simulink model "heli_q8"  (R2015b)
settings: Solver=ode1  StartTime=0.0  StopTime=inf  FixedStep=0.002  RelTol=1e-3
PostLoadFcn:
  | qc_set_target_type(getConfigSet(bdroot, 'QUARC Default Target Configuration'));
values from neighbouring files (symbols this model uses):
  F_aug = inv(C*inv(B*K_aug_K1-A)*B)    [init_heli.m]
  Joystick_gain_x = 1    [init_heli.m]
  Joystick_gain_y = 1    [init_heli.m]
  k_1 = k_f/(2*m_p*l_p)    (= 0.514757969303)    [init_heli.m]
  k_2 = (l_h*k_f)/(m_c*l_c^2+2*m_p*l_h^2)    (= 0.0828365392735)    [init_heli.m]
  k_3 = (v_s0*l_h*k_f)/(m_c*l_c^2+2*m_p*(l_h^2+l_p^2))    (= 0.611739028763)    [init_heli.m]
  K_aug = lqr(A_aug,B_aug,Q_aug,R_aug)    [init_heli.m]
  k_pd = (2*zeta*omega_0)/k_1    (= 7.77064220183)    [init_heli.m]
  k_pp = omega_0^2/k_1    (= 7.77064220183)    [init_heli.m]
  v_s0 = 7.7    [init_heli.m]
undefined symbols (not defined in the file or in its folder): HIL, qc_get_step_size
libraries: quarc_library x4, simulink x1
settings Model: SimulationMode=external  ExtModeTrigDuration=5000  Creator=Rchan  LastModifiedBy=torsteoe
settings SolverCC: PositivePriorityOrder=on
settings DataIOCC: SaveFormat=Array  SignalLoggingSaveFormat=ModelDataLogs
settings OptimizationCC: ExpressionDepthLimit=2147483647  InitFltsAndDblsToZero=on
settings DebuggingCC: SaveWithParameterizedLinksMsg=none  UnderspecifiedInitializationDetection=Classic  MergeDetectMultiDrivingBlocksExec=none  SolverPrmCheckMsg=warning  MultiTaskDSMMsg=warning  MultiTaskCondExecSysMsg=none  FcnCallInpInsideContextMsg=UseLocalSettings  StateNameClashWarn=warning
settings HardwareCC: ProdBitPerPointer=32  ProdLargestAtomicFloat=None  ProdIntDivRoundTo=Undefined  ProdEndianess=Unspecified  ProdWordSize=32  ProdHWDeviceType=32-bit Generic
settings RTWCC: SystemTargetFile=quarc_win64.tlc  TemplateMakefile=quarc_default_tmf  Description=QUARC Win64 Target
settings GRTTargetCC: ParMdlRefBuildCompliant=off  CompOptLevelCompliant=off  GeneratePreprocessorConditionals=Disable all  CombineOutputUpdateFcns=off  MatFileLogging=off  GRTInterface=on  UseToolchainInfoCompliant=off  ExtMode=on  ExtModeMexFile=quarc_comm
settings ConfigComp: CovModelRefEnable=Off  CovSFcnEnable=off

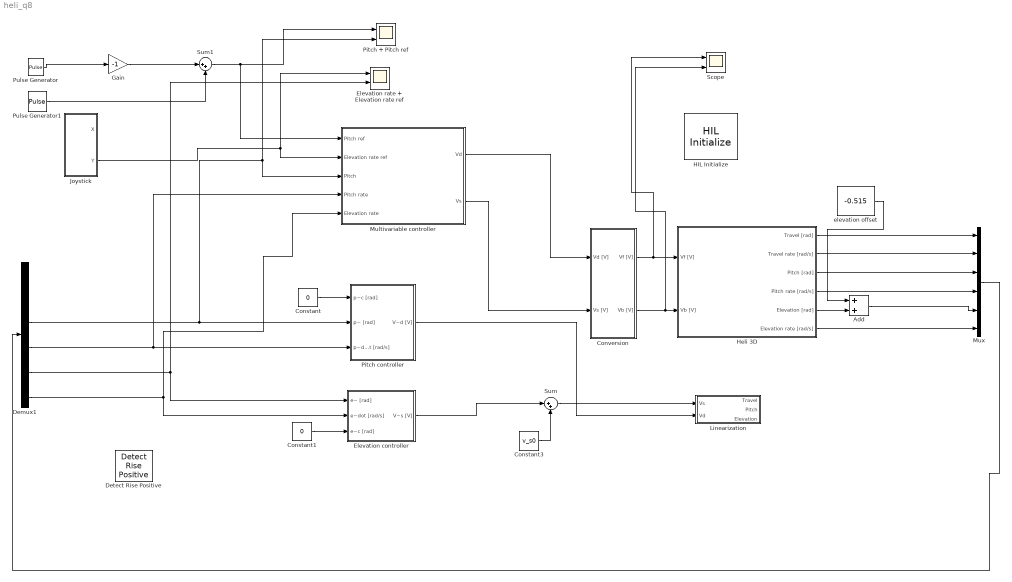
== system heli_q8 ==
  Add : Sum
  Constant : Constant  Value=0
  Constant1 : Constant  Value=0
  Constant3 : Constant  Value=v_s0
  Conversion : Subsystem
  Demux1 : Demux  Outputs=6
  Detect Rise Positive : simulink/Logic and Bit Operations/Detect Rise Positive  vinit=0  InputProcessing=Inherited  OutDataTypeStr=boolean
  Elevation controller : Subsystem
  Elevation rate + Elevation rate ref : Scope  NumInputPorts=2
  Gain : Gain  Gain=-1
  HIL Initialize : quarc_library/Data Acquisition/Generic/Configuration/HIL Initialize  Priority=-99  object_name=HIL-1  board_type=q8_usb  board_number=0  board_options=update_rate=normal;decimation=1  exclusive=off  active=off  hardware_clocks=[0:2]  clock_modes=[]  initial_clock_frequencies=[]  set_clock_params_at_start=off  set_clock_params_at_switch_in=off  set_clock_frequencies_at_start=off  set_clock_frequencies_at_switch_in=off  analog_input_channels=[0:7]  analog_input_maximums=10  analog_input_minimums=-10  set_analog_input_params_at_start=on  set_analog_input_params_at_switch_in=off  analog_output_channels=[0:7]  analog_output_maximums=10  analog_output_minimums=-10  initial_analog_outputs=[0]  final_analog_outputs=[0]  watchdog_analog_outputs=0  set_analog_output_params_at_start=on  set_analog_output_params_at_switch_in=off  set_analog_outputs_at_start=on  set_analog_outputs_at_switch_in=off  set_analog_outputs_at_terminate=on  set_analog_outputs_at_switch_out=off  set_analog_outputs_on_watchdog=off  digital_input_channels=[]  digital_output_channels=[]  digital_output_configuration=[]  initial_digital_outputs=[1]  final_digital_outputs=[1]  watchdog_digital_outputs=[1]  set_digital_output_params_at_start=off  set_digital_output_params_at_switch_in=off  set_digital_outputs_at_start=on  set_digital_outputs_at_switch_in=off  set_digital_outputs_at_terminate=on  set_digital_outputs_at_switch_out=off  set_digital_outputs_on_watchdog=off  encoder_channels=[0:7]  quadrature=[4]  encoder_filter_frequency=[]  initial_encoder_counts=[0]  set_encoder_params_at_start=on  set_encoder_params_at_switch_in=off  set_encoder_counts_at_start=on  set_encoder_counts_at_switch_in=off  pwm_channels=[0:7]  pwm_modes=0  pwm_frequency=99.532799999999995e6/4095  pwm_configuration=[0]  pwm_alignment=[0]  pwm_polarity=[1]  pwm_leading_deadband=[0]  pwm_trailing_deadband=[0]  initial_pwm_outputs=[0]  final_pwm_outputs=[0]  watchdog_pwm_outputs=[0]  set_pwm_params_at_start=on  set_pwm_params_at_switch_in=off  set_pwm_outputs_at_start=on  set_pwm_outputs_at_switch_in=off  set_pwm_outputs_at_terminate=on  set_pwm_outputs_at_switch_out=off  set_pwm_outputs_on_watchdog=off  other_output_channels=[]  initial_other_outputs=[]  final_other_outputs=[]  watchdog_other_outputs=[]  set_other_outputs_at_start=off  set_other_outputs_at_switch_in=off  set_other_outputs_at_terminate=off  set_other_outputs_at_switch_out=off  set_other_outputs_on_watchdog=off
  Heli 3D : Subsystem
  Joystick : Subsystem
  Linearization : Subsystem
  Multivariable controller : Subsystem
  Mux : Mux  Inputs=6
  Pitch + Pitch ref : Scope  NumInputPorts=2
  Pitch controller : Subsystem
  Pulse Generator : DiscretePulseGenerator  PulseType=Time based  Amplitude=0.5  Period=40  PulseWidth=50  PhaseDelay=10
  Pulse Generator1 : DiscretePulseGenerator  PulseType=Time based  Amplitude=0.5  Period=40  PulseWidth=50  PhaseDelay=30
  Scope : Scope  NumInputPorts=2
  Sum : Sum  Inputs=|++
  Sum1 : Sum  Inputs=|++
  elevation offset : Constant  Value=-0.515
  wires:
  Conversion/1(Vf [V]) -> Scope/1, Heli 3D/1(Vf [V])
  Heli 3D/1(Travel [rad]) -> Mux/1
  Heli 3D/2(Travel rate [rad/s]) -> Mux/2
  Heli 3D/3(Pitch [rad]) -> Mux/3
  Heli 3D/4(Pitch rate [rad/s]) -> Mux/4
  Heli 3D/5(Elevation [rad]) -> Add/2
  Heli 3D/6(Elevation rate [rad/s]) -> Mux/6
  Add/1 -> Mux/5
  elevation offset/1 -> Add/1
  Conversion/2(Vb [V]) -> Scope/2, Heli 3D/2(Vb [V])
  Constant/1 -> Pitch controller/1(p~c [rad])
  Constant1/1 -> Elevation controller/3(e~c [rad])
  Elevation controller/1(V~s [V]) -> Sum/1
  Sum/1 -> Linearization/1("Vs ")
  Pitch controller/1(V~d [V]) -> Linearization/2("Vd ")
  Joystick/2(Y) -> Elevation rate + Elevation rate ref/1, Multivariable controller/2(Elevation rate ref)
  Constant3/1 -> Sum/2
  Mux/1 -> Demux1/1
  Demux1/3 -> Pitch + Pitch ref/2, Multivariable controller/3(Pitch), Pitch controller/2(p~ [rad])
  Demux1/4 -> Multivariable controller/4(Pitch rate), Pitch controller/3(p~dot [rad/s])
  Demux1/5 -> Elevation controller/1(e~ [rad]), Elevation rate + Elevation rate ref/2
  Multivariable controller/1(Vd) -> Conversion/1(Vd [V])
  Pulse Generator/1 -> Gain/1
  Pulse Generator1/1 -> Sum1/2
  Gain/1 -> Sum1/1
  Multivariable controller/2(Vs) -> Conversion/2(Vs [V])
  Sum1/1 -> Multivariable controller/1("Pitch ref "), Pitch + Pitch ref/1
  Demux1/6 -> Multivariable controller/5(Elevation rate), Elevation controller/2(e~dot [rad/s])

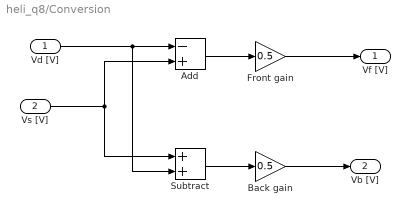
== system heli_q8/Conversion ==
  Vd [V] : Inport
  Vs [V] : Inport  Port=2
  Add : Sum  Inputs=-+
  Back gain : Gain  Gain=0.5
  Front gain : Gain  Gain=0.5
  Subtract : Sum
  Vf [V] : Outport
  Vb [V] : Outport  Port=2
  wires:
  Vd [V]/1 -> Subtract/2, Add/1
  Vs [V]/1 -> Subtract/1, Add/2
  Subtract/1 -> Back gain/1
  Back gain/1 -> Vb [V]/1
  Add/1 -> Front gain/1
  Front gain/1 -> Vf [V]/1

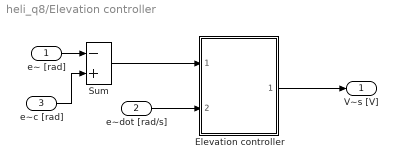
== system heli_q8/Elevation controller ==
  e~ [rad] : Inport
  e~dot [rad/s] : Inport  Port=2
  e~c [rad] : Inport  Port=3
  Elevation controller : Subsystem
  Sum : Sum  Inputs=-+  SaturateOnIntegerOverflow=on  InputSameDT=on  OutDataTypeStr=Inherit: Same as first input
  V~s [V] : Outport  InitialOutput=0
  wires:
  Sum/1 -> Elevation controller/1(e~ [rad])
  Elevation controller/1(V~_s [V]) -> V~s [V]/1
  e~ [rad]/1 -> Sum/1
  e~dot [rad/s]/1 -> Elevation controller/2(e~_dot [rad/s])
  e~c [rad]/1 -> Sum/2

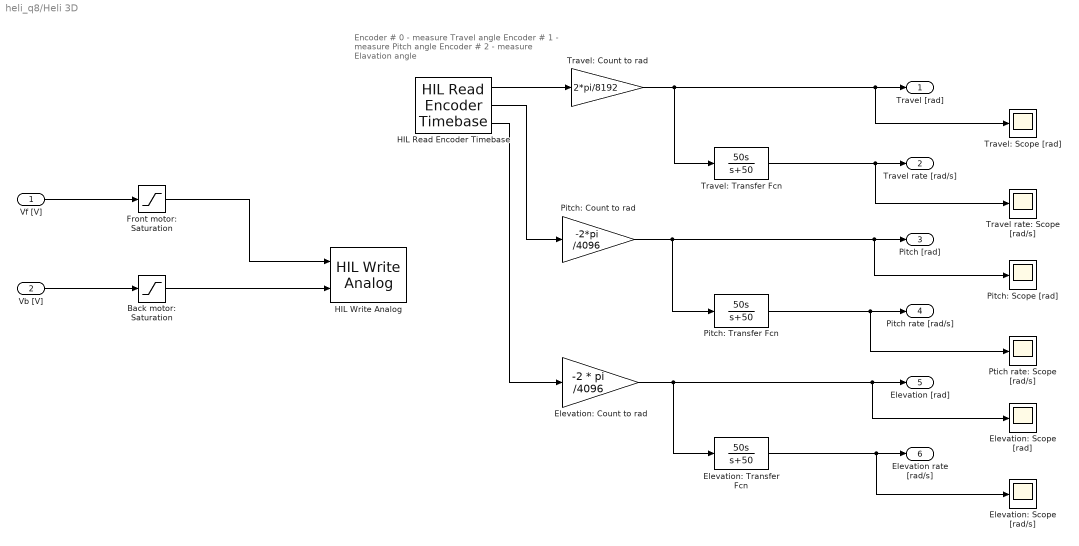
== system heli_q8/Heli 3D ==
  note: Encoder # 0 - measure Travel angle
      | Encoder # 1 - measure Pitch angle
      | Encoder # 2 - measure Elavation angle
  Vf [V] : Inport
  Vb [V] : Inport  Port=2
  Back motor: Saturation : Saturate  UpperLimit=5  LowerLimit=-5
  Elevation: Count to rad : Gain  Gain=-2 * pi /4096
  Elevation: Scope [rad/s] : Scope
  Elevation: Scope [rad] : Scope
  Elevation: Transfer Fcn : TransferFcn  Numerator=[50 0]  Denominator=[1 50]
  Front motor: Saturation : Saturate  UpperLimit=5  LowerLimit=-5
  HIL Read Encoder Timebase : quarc_library/Data Acquisition/Generic/Timebases/HIL Read Encoder Timebase  object_name=HIL-1  clock=0  channels=[0:2]  samples_in_buffer=max(ceil(1/qc_get_step_size), 1)  active=on  vector_output=off  data_type_mode=Inherit via back propagation  data_type=double
  HIL Write Analog : quarc_library/Data Acquisition/Generic/Immediate I//O/HIL Write Analog  object_name=HIL-1  channels=[0:1]  sample_time=-1  active=off  vector_input=off
  Pitch: Count to rad : Gain  Gain=-2*pi /4096
  Pitch: Scope [rad] : Scope
  Pitch: Transfer Fcn : TransferFcn  Numerator=[50 0]  Denominator=[1 50]
  Ptich rate: Scope [rad/s] : Scope
  Travel rate: Scope [rad/s] : Scope
  Travel: Count to rad : Gain  Gain=2*pi/8192
  Travel: Scope [rad] : Scope
  Travel: Transfer Fcn : TransferFcn  Numerator=[50 0]  Denominator=[1 50]
  Travel [rad] : Outport
  Travel rate [rad/s] : Outport  Port=2
  Pitch [rad] : Outport  Port=3
  Pitch rate [rad/s] : Outport  Port=4
  Elevation [rad] : Outport  Port=5
  Elevation rate [rad/s] : Outport  Port=6
  wires:
  HIL Read Encoder Timebase/1 -> Travel: Count to rad/1
  HIL Read Encoder Timebase/2 -> Pitch: Count to rad/1
  HIL Read Encoder Timebase/3 -> Elevation: Count to rad/1
  Travel: Count to rad/1 -> Travel: Scope [rad]/1, Travel [rad]/1, Travel: Transfer Fcn/1
  Travel: Transfer Fcn/1 -> Travel rate: Scope [rad/s]/1, Travel rate [rad/s]/1
  Pitch: Count to rad/1 -> Pitch: Transfer Fcn/1, Pitch: Scope [rad]/1, Pitch [rad]/1
  Pitch: Transfer Fcn/1 -> Ptich rate: Scope [rad/s]/1, Pitch rate [rad/s]/1
  Elevation: Count to rad/1 -> Elevation: Transfer Fcn/1, Elevation: Scope [rad]/1, Elevation [rad]/1
  Elevation: Transfer Fcn/1 -> Elevation: Scope [rad/s]/1, Elevation rate [rad/s]/1
  Vf [V]/1 -> Front motor: Saturation/1
  Vb [V]/1 -> Back motor: Saturation/1
  Front motor: Saturation/1 -> HIL Write Analog/1
  Back motor: Saturation/1 -> HIL Write Analog/2

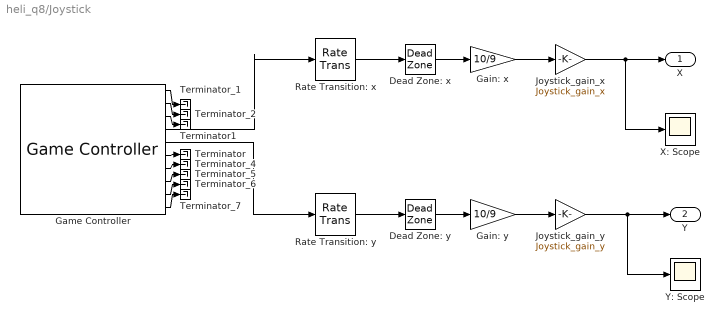
== system heli_q8/Joystick ==
  Dead Zone: x : DeadZone  LowerValue=-0.1  UpperValue=0.1  SaturateOnIntegerOverflow=on
  Dead Zone: y : DeadZone  LowerValue=-0.1  UpperValue=0.1  SaturateOnIntegerOverflow=on
  Gain: x : Gain  Gain=10/9
  Gain: y : Gain  Gain=10/9
  Game Controller : quarc_library/Devices/Peripherals/Target/Game Controller  controller=1  buffer_size=12  deadzone=[]  saturation=[]  sample_time=max(qc_get_step_size, 0.01)  auto_center=off  enabled=on
  Joystick_gain_x : Gain  Gain=Joystick_gain_x
  Joystick_gain_y : Gain  Gain=Joystick_gain_y
  Rate Transition: x : RateTransition
  Rate Transition: y : RateTransition
  Terminator : Terminator
  Terminator1 : Terminator
  Terminator_{1..2,4..7} (6 alike) : Terminator
  X: Scope : Scope
  Y: Scope : Scope
  X : Outport
  Y : Outport  Port=2
  wires:
  Rate Transition: y/1 -> Dead Zone: y/1
  Rate Transition: x/1 -> Dead Zone: x/1
  Game Controller/5 -> Rate Transition: y/1
  Game Controller/4 -> Rate Transition: x/1
  Game Controller/1 -> Terminator_1/1
  Game Controller/2 -> Terminator_2/1
  Game Controller/7 -> Terminator_4/1
  Game Controller/8 -> Terminator_5/1
  Game Controller/9 -> Terminator_6/1
  Game Controller/10 -> Terminator_7/1
  Game Controller/3 -> Terminator1/1
  Game Controller/6 -> Terminator/1
  Dead Zone: x/1 -> Gain: x/1
  Dead Zone: y/1 -> Gain: y/1
  Gain: x/1 -> Joystick_gain_x/1
  Gain: y/1 -> Joystick_gain_y/1
  Joystick_gain_x/1 -> X/1, X: Scope/1
  Joystick_gain_y/1 -> Y: Scope/1, Y/1

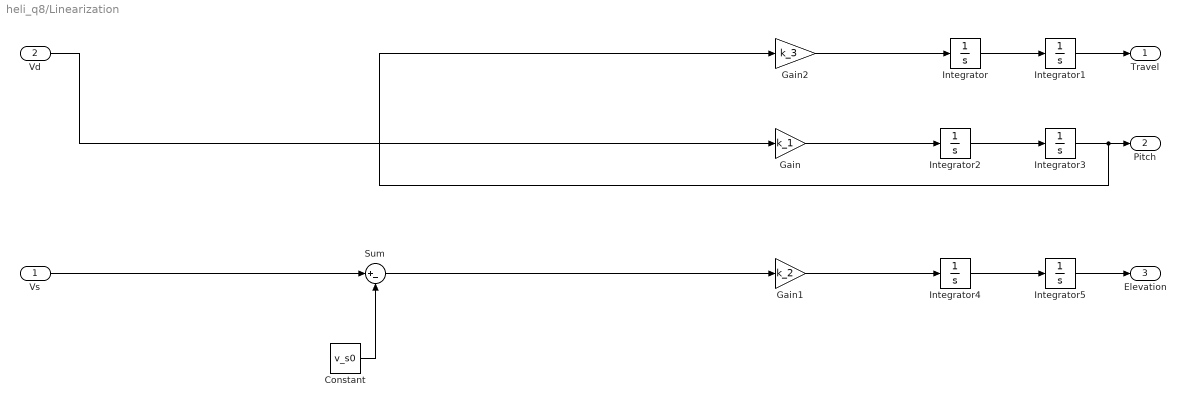
== system heli_q8/Linearization ==
  "Vs " : Inport
  "Vd " : Inport  Port=2
  Constant : Constant  Value=v_s0
  Gain : Gain  Gain=k_1
  Gain1 : Gain  Gain=k_2
  Gain2 : Gain  Gain=k_3
  Integrator{,1..5} (6 alike) : Integrator
  Sum : Sum  Inputs=|+-
  Travel : Outport
  Pitch : Outport  Port=2
  Elevation : Outport  Port=3
  wires:
  Integrator5/1 -> Elevation/1
  Integrator4/1 -> Integrator5/1
  Integrator2/1 -> Integrator3/1
  Integrator1/1 -> Travel/1
  Integrator/1 -> Integrator1/1
  Gain/1 -> Integrator2/1
  Gain1/1 -> Integrator4/1
  Gain2/1 -> Integrator/1
  Integrator3/1 -> Gain2/1, Pitch/1
  "Vd "/1 -> Gain/1
  "Vs "/1 -> Sum/1
  Sum/1 -> Gain1/1
  Constant/1 -> Sum/2

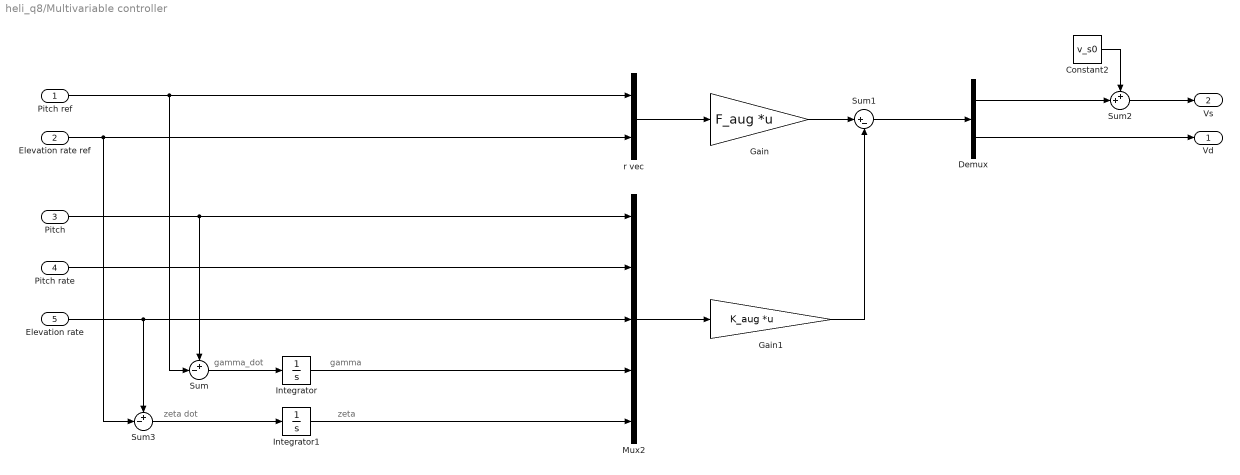
== system heli_q8/Multivariable controller ==
  note: zeta
  note: zeta dot
  note: gamma
  note: gamma_dot
  "Pitch ref " : Inport
  Elevation rate ref : Inport  Port=2
  Pitch : Inport  Port=3
  Pitch rate : Inport  Port=4
  Elevation rate : Inport  Port=5
  Constant2 : Constant  Value=v_s0
  Demux : Demux  Outputs=2
  Gain : Gain  Gain=F_aug  Multiplication=Matrix(K*u) (u vector)
  Gain1 : Gain  Gain=K_aug  Multiplication=Matrix(K*u) (u vector)
  Integrator : Integrator
  Integrator1 : Integrator
  Mux2 : Mux  Inputs=5
  Sum : Sum  Inputs=+-|
  Sum1 : Sum  Inputs=|+-
  Sum2 : Sum  Inputs=++|
  Sum3 : Sum  Inputs=+-|
  r vec : Mux  Inputs=2
  Vd : Outport
  Vs : Outport  Port=2
  wires:
  r vec/1 -> Gain/1
  Elevation rate ref/1 -> Sum3/2, r vec/2
  Gain/1 -> Sum1/1
  Mux2/1 -> Gain1/1
  Gain1/1 -> Sum1/2
  Elevation rate/1 -> Mux2/3, Sum3/1
  Pitch/1 -> Sum/1, Mux2/1
  Pitch rate/1 -> Mux2/2
  Constant2/1 -> Sum2/1
  Demux/2 -> Vd/1
  Sum2/1 -> Vs/1
  Sum1/1 -> Demux/1
  Demux/1 -> Sum2/2
  "Pitch ref "/1 -> Sum/2, r vec/1
  Sum/1 -> Integrator/1
  Sum3/1 -> Integrator1/1
  Integrator/1 -> Mux2/4
  Integrator1/1 -> Mux2/5

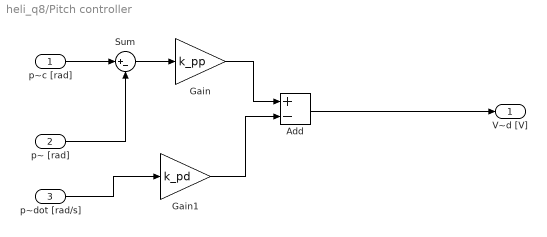
== system heli_q8/Pitch controller ==
  p~c [rad] : Inport
  p~ [rad] : Inport  Port=2
  p~dot [rad/s] : Inport  Port=3
  Add : Sum  Inputs=+-
  Gain : Gain  Gain=k_pp
  Gain1 : Gain  Gain=k_pd
  Sum : Sum  Inputs=|+-
  V~d [V] : Outport  InitialOutput=0
  wires:
  p~c [rad]/1 -> Sum/1
  p~ [rad]/1 -> Sum/2
  Sum/1 -> Gain/1
  Gain/1 -> Add/1
  Gain1/1 -> Add/2
  p~dot [rad/s]/1 -> Gain1/1
  Add/1 -> V~d [V]/1

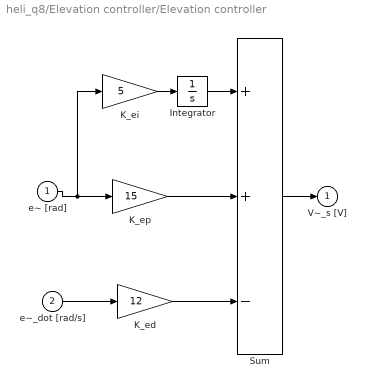
== system heli_q8/Elevation controller/Elevation controller ==
  e~ [rad] : Inport
  e~_dot [rad/s] : Inport  Port=2
  Integrator : Integrator  LimitOutput=on
  K_ed : Gain  Gain=12  SaturateOnIntegerOverflow=on  OutDataTypeStr=Inherit: Same as input  ParamDataTypeStr=Inherit: Same as input
  K_ei : Gain  Gain=5  SaturateOnIntegerOverflow=on  OutDataTypeStr=Inherit: Same as input  ParamDataTypeStr=Inherit: Same as input
  K_ep : Gain  Gain=15  SaturateOnIntegerOverflow=on  OutDataTypeStr=Inherit: Same as input  ParamDataTypeStr=Inherit: Same as input
  Sum : Sum  Inputs=++-  SaturateOnIntegerOverflow=on  InputSameDT=on  OutDataTypeStr=Inherit: Same as first input
  V~_s [V] : Outport  InitialOutput=0
  wires:
  K_ei/1 -> Integrator/1
  Integrator/1 -> Sum/1
  Sum/1 -> V~_s [V]/1
  e~_dot [rad/s]/1 -> K_ed/1
  K_ed/1 -> Sum/3
  K_ep/1 -> Sum/2
  e~ [rad]/1 -> K_ep/1, K_ei/1
